simulink model "tank_flow_test"  (R2020a)
settings: Solver=VariableStepAuto  StartTime=0.0  StopTime=100  RelTol=1e-3  AbsTol=1e-3
libraries: nesl_utility x5, sh_lib x4
settings Model: Creator=Afraz  LastModifiedBy=Afraz
settings SolverCC: AutoScaleAbsTol=off
settings DebuggingCC: SymbolicDimsDataTypeCodeGenerationDiagnostic=none
settings SFSimCC: CustomCodeUndefinedFunction=UseInterfaceOnly
settings SimscapeCC: SimscapeLogType=all  SimscapeLogSimulationStatistics=on  SimscapeLogDataHistory=10000

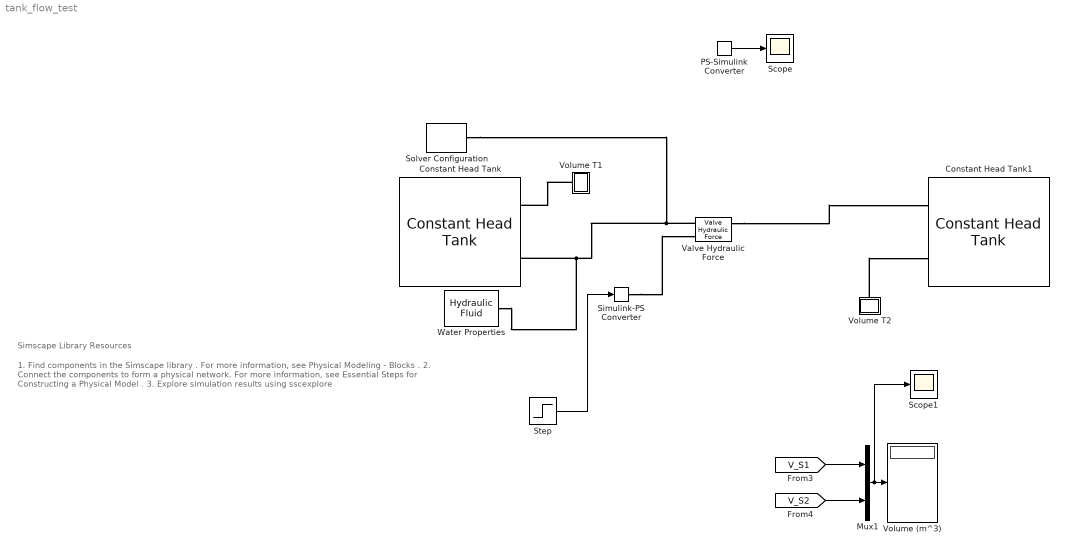
== system tank_flow_test ==
  note: 1. Find components in the Simscape library .
      | For more information, see Physical Modeling - Blocks .
      | 2. Connect the components to form a physical network.
      | For more information, see Essential Steps for Constructing a Physical Model .
      | 3. Explore simulation results using sscexplore
  note: Simscape Library Resources
  Constant Head Tank : sh_lib/Low-Pressure Blocks/Constant Head Tank  press=10 bar  fluid_level=1 m  pipe_diam=0.02 m  loss_coeff=1.2  g=9.80665 m/s^2  volume_specify=on  volume_priority=High  volume=.2 m^3  volume_nominal_specify=off  volume_nominal_unit=m^3  volume_nominal_value=1
      settings: SourceProductBaseCode=SH  InternalSimscapePortConfiguration="{\"Bottom\":[],\"Left\":[],\"Right\":[{\"id\":\"V\",\"label\":\"V\",\"type\":\"output\"},{\"id\":\"T\",\"label\":\"T\",\"type\":\"foundation.hydraulic.hydraulic\"}],\"Top\":[]}"
  Constant Head Tank1 : sh_lib/Low-Pressure Blocks/Constant Head Tank  press=1 bar  fluid_level=1 m  pipe_diam=0.02 m  loss_coeff=1.2  g=9.80665 m/s^2  volume_specify=off  volume_priority=High  volume=0.2 m^3  volume_nominal_specify=off  volume_nominal_unit=m^3  volume_nominal_value=1
      settings: SourceProductBaseCode=SH  InternalSimscapePortConfiguration="{\"Bottom\":[],\"Left\":[],\"Right\":[{\"id\":\"V\",\"label\":\"V\",\"type\":\"output\"},{\"id\":\"T\",\"label\":\"T\",\"type\":\"foundation.hydraulic.hydraulic\"}],\"Top\":[]}"
  Mux1 : Mux  Inputs=2
  PS-Simulink Converter : nesl_utility/PS-Simulink Converter  PhysicalDomain=network_engine_domain  SubClassName=ps_output  LeftPortType=input  RightPortType=output  PseudoPeriodic=off  Frequencies=[]  Unit=inherit  AffineConversion=off
      settings: SourceProductBaseCode=MT,SS
  Scope : Scope
  Scope1 : Scope
  Simulink-PS Converter : nesl_utility/Simulink-PS Converter  PhysicalDomain=network_engine_domain  SubClassName=ps_input  LeftPortType=input  RightPortType=output  PseudoPeriodic=off  Frequencies=[]  NoiseDistribution=none  NoiseParameters=[]  Unit=1  AffineConversion=off  FilteringAndDerivatives=provide  SimscapeFilterOrder=1  InputFilterTimeConstant=0.001  UdotUserProvided=0
      settings: SourceProductBaseCode=MT,SS
  Solver Configuration : nesl_utility/Solver Configuration  PhysicalDomain=network_engine_domain  SubClassName=solver  LeftPortType=input  RightPortType=generic  Tones=[]  Harmonics=[]  SimulateNoise=off  Profile=off  UseLocalSampling=off  EnableSwitchedLinearOptims=on  FrequencyDomain=off  UseCCode=off  RelTol=0.001  AbsTol=1e-06  MinStep=1e-09  ToWorkspace=off  RevertToSquareIcSolve=off  NumHomotopyIterations=100  PhasorMode=off  PhasorModeNumHarmonics=1  DoDC=off  ResidualTolerance=1e-09  UseLocalSolver=off  LocalSolverChoice=NE_BACKWARD_EULER_ADVANCER  LocalSolverSampleTime=0.001  DoFixedCost=off  MaxNonlinIter=3  MaxModeIter=2  LinearAlgebra=auto  EquationFormulation=NE_TIME_EF  DelaysMemoryBudget=1024  AutomaticFiltering=on  FilteringTimeConstant=0.001  PartitionStorageMethod=AS_NEEDED  PartitionMemoryBudget=1024  PartitionMethod=ROBUST
      settings: SourceProductBaseCode=MT,SS
  Step : Step  Time=20  SampleTime=0
  Valve Hydraulic Force : sh_lib/Valves/Valve Forces/Valve Hydraulic Force  x_0=0 m  or=1  opening_tab=[0, .001, .002, .003, .004] m  pressure_tab=[-10000000, -7500000, -5000000, -2500000, 0, 2500000, 5000000, 7500000, 10000000] Pa  force_tab=[0, -127.3576, -27.8944, 227.2513, 575.3104; 0, -95.5182, -20.9208, 170.4385, 431.4828; 0, -63.6788, -13.9472, 113.6256, 287.6552; 0, -31.8394, -6.9736, 56.8128, 143.8276; 0, 0, 0, 0, 0; 196.3495, 120.7506, 97.5709, 111.9898, 150.9306; 392.6991, 241.5013, 195.1418, 223.9797, 301.8613; 589.0486, 362.2519, 292.7126, 335.9695, 452.7919; 785.3982, 483.0025, 390.2835, 447.9594, 603.7225] N  interp_method=simscape.enum.interpolation.linear  extrap_method=simscape.enum.extrapolation.linear
      settings: SourceProductBaseCode=SH  InternalSimscapePortConfiguration="{\"Bottom\":[],\"Left\":[{\"id\":\"A\",\"label\":\"A\",\"type\":\"foundation.hydraulic.hydraulic\"},{\"id\":\"S\",\"label\":\"S\",\"type\":\"input\"}],\"Right\":[{\"id\":\"B\",\"label\":\"B\",\"type\":\"foundation.hydraulic.hydraulic\"},{\"id\":\"F\",\"label\":\"F\",\"type\":\"output\"}],\"Top\":[]}"
  Volume (m^3) : Display
  Volume T1 : Subsystem
  Volume T2 : Subsystem
  Water Properties : sh_lib/Hydraulic Utilities/Hydraulic Fluid  DataSource=1  SelFluid=24  SysTemp=1  TrapAir=0.001  ViscDerFactor=1  range_error=2
  wires:
  PS-Simulink Converter/1 -> Scope/1
  Step/1 -> Simulink-PS Converter/1
  [V_S1] -> Mux1/1
  Mux1/1 -> Scope1/1, Volume (m^3)/1
  [V_S2] -> Mux1/2
  connections:
  Simulink-PS Converter/RConn1 -- Valve Hydraulic Force/LConn2
  Valve Hydraulic Force/LConn1 -- Solver Configuration/RConn1 -- Water Properties/RConn1 -- Constant Head Tank/RConn2
  Valve Hydraulic Force/RConn1 -- Constant Head Tank1/RConn2
  Volume T1/LConn1 -- Constant Head Tank/RConn1
  Volume T2/LConn1 -- Constant Head Tank1/RConn1

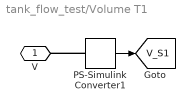
== system tank_flow_test/Volume T1 ==
  PS-Simulink Converter1 : nesl_utility/PS-Simulink Converter  PhysicalDomain=network_engine_domain  SubClassName=ps_output  LeftPortType=input  RightPortType=output  PseudoPeriodic=off  Frequencies=[]  Unit=1  AffineConversion=off
      settings: SourceProductBaseCode=MT,SS
  V : PMIOPort  Side=Left
  tag scope: V_S1=global
  wires:
  PS-Simulink Converter1/1 -> [V_S1]
  connections:
  PS-Simulink Converter1/LConn1 -- V/RConn1

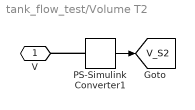
== system tank_flow_test/Volume T2 ==
  PS-Simulink Converter1 : nesl_utility/PS-Simulink Converter  PhysicalDomain=network_engine_domain  SubClassName=ps_output  LeftPortType=input  RightPortType=output  PseudoPeriodic=off  Frequencies=[]  Unit=1  AffineConversion=off
      settings: SourceProductBaseCode=MT,SS
  V : PMIOPort  Side=Left
  tag scope: V_S2=global
  wires:
  PS-Simulink Converter1/1 -> [V_S2]
  connections:
  PS-Simulink Converter1/LConn1 -- V/RConn1
